simulink model "Task4"  (R2013b)
settings: Solver=ode45  StartTime=0.0  StopTime=1.0  RelTol=1e-3
settings Model: Creator=barnetdavi  LastModifiedBy=barnetdavi

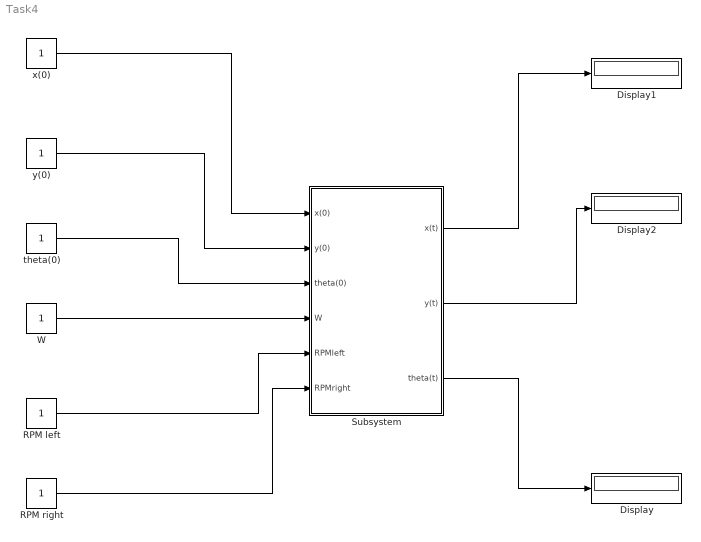
== system Task4 ==
  Display : Display
  Display1 : Display
  Display2 : Display
  RPM left : Constant
  RPM right : Constant
  Subsystem : Subsystem
  W : Constant
  theta(0) : Constant
  x(0) : Constant
  y(0) : Constant
  wires:
  x(0)/1 -> Subsystem/1(x(0))
  y(0)/1 -> Subsystem/2(y(0))
  theta(0)/1 -> Subsystem/3(theta(0))
  W/1 -> Subsystem/4(W)
  RPM left/1 -> Subsystem/5(RPMleft)
  RPM right/1 -> Subsystem/6(RPMright)
  Subsystem/1(x(t)) -> Display1/1
  Subsystem/2(y(t)) -> Display2/1
  Subsystem/3(theta(t)) -> Display/1

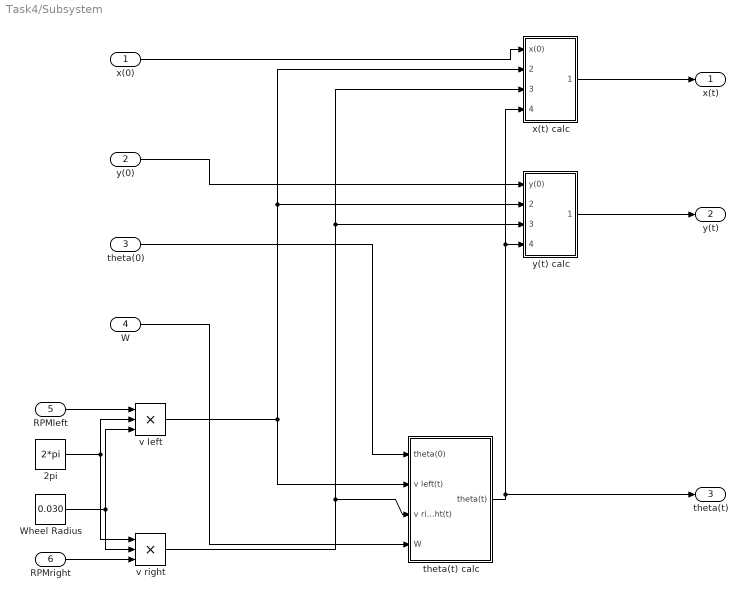
== system Task4/Subsystem ==
  x(0) : Inport
  y(0) : Inport  Port=2
  theta(0) : Inport  Port=3
  W : Inport  Port=4
  RPMleft : Inport  Port=5
  RPMright : Inport  Port=6
  2pi : Constant  Value=2*pi
  Wheel Radius : Constant  Value=0.030
  theta(t) calc : Subsystem
  v left : Product  Inputs=3
  v right : Product  Inputs=3
  x(t) calc : Subsystem
  y(t) calc : Subsystem
  x(t) : Outport
  y(t) : Outport  Port=2
  theta(t) : Outport  Port=3
  wires:
  x(t) calc/1(Out1) -> x(t)/1
  theta(t) calc/1(theta(t)) -> theta(t)/1, y(t) calc/4(theta(t)), x(t) calc/4(theta(t))
  v left/1 -> x(t) calc/2(v left), y(t) calc/2(V left), theta(t) calc/2(v left(t))
  y(0)/1 -> y(t) calc/1(y(0))
  theta(0)/1 -> theta(t) calc/1(theta(0))
  v right/1 -> x(t) calc/3(v right), y(t) calc/3(V right), theta(t) calc/3(v right(t))
  x(0)/1 -> x(t) calc/1(x(0))
  W/1 -> theta(t) calc/4(W)
  y(t) calc/1(Out1) -> y(t)/1
  RPMleft/1 -> v left/1
  2pi/1 -> v right/1, v left/2
  Wheel Radius/1 -> v right/2, v left/3
  RPMright/1 -> v right/3

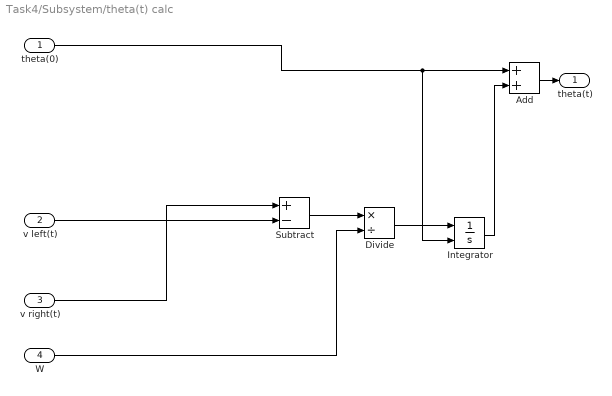
== system Task4/Subsystem/theta(t) calc ==
  theta(0) : Inport
  v left(t) : Inport  Port=2
  v right(t) : Inport  Port=3
  W : Inport  Port=4
  Add : Sum
  Divide : Product  Inputs=*/
  Integrator : Integrator  InitialConditionSource=external
  Subtract : Sum  Inputs=+-
  theta(t) : Outport
  wires:
  Subtract/1 -> Divide/1
  Divide/1 -> Integrator/1
  Integrator/1 -> Add/2
  theta(0)/1 -> Integrator/2, Add/1
  Add/1 -> theta(t)/1
  v right(t)/1 -> Subtract/1
  v left(t)/1 -> Subtract/2
  W/1 -> Divide/2

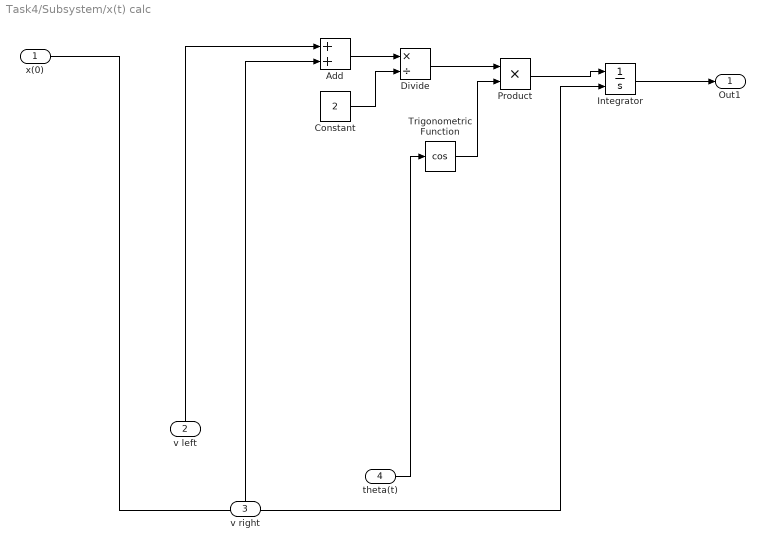
== system Task4/Subsystem/x(t) calc ==
  x(0) : Inport
  v left : Inport  Port=2
  v right : Inport  Port=3
  theta(t) : Inport  Port=4
  Add : Sum
  Constant : Constant  Value=2
  Divide : Product  Inputs=*/
  Integrator : Integrator  InitialConditionSource=external
  Product : Product
  Trigonometric Function : Trigonometry  Operator=cos
  Out1 : Outport
  wires:
  Constant/1 -> Divide/2
  theta(t)/1 -> Trigonometric Function/1
  v right/1 -> Add/2
  Product/1 -> Integrator/1
  Divide/1 -> Product/1
  v left/1 -> Add/1
  x(0)/1 -> Integrator/2
  Add/1 -> Divide/1
  Integrator/1 -> Out1/1
  Trigonometric Function/1 -> Product/2

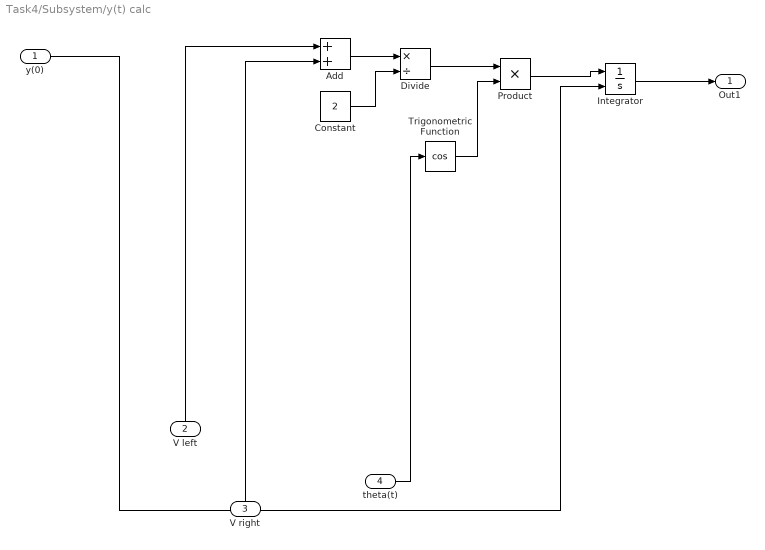
== system Task4/Subsystem/y(t) calc ==
  y(0) : Inport
  V left : Inport  Port=2
  V right : Inport  Port=3
  theta(t) : Inport  Port=4
  Add : Sum
  Constant : Constant  Value=2
  Divide : Product  Inputs=*/
  Integrator : Integrator  InitialConditionSource=external
  Product : Product
  Trigonometric Function : Trigonometry  Operator=cos
  Out1 : Outport
  wires:
  Constant/1 -> Divide/2
  theta(t)/1 -> Trigonometric Function/1
  V right/1 -> Add/2
  Product/1 -> Integrator/1
  Divide/1 -> Product/1
  V left/1 -> Add/1
  y(0)/1 -> Integrator/2
  Add/1 -> Divide/1
  Integrator/1 -> Out1/1
  Trigonometric Function/1 -> Product/2
